simulink model "untitled"  (R2025a)
settings: Solver=VariableStepAuto  StartTime=0.0  StopTime=0.2  RelTol=1e-3
settings Model: Creator=vm66c  LastModifiedBy=vm66c

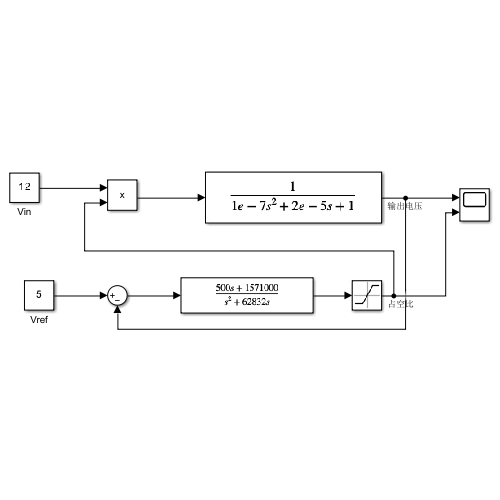
[thumbnail: Simulink's stored preview of the top-level diagram]
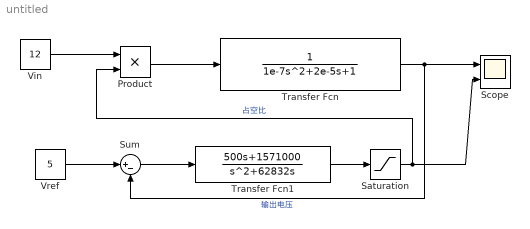
== system untitled ==
  Product : Product
  Saturation : Saturate  UpperLimit=0.9  LowerLimit=0.1
  Scope : Scope  NumInputPorts=2
      settings: ActiveDisplayYMinimum=-70.471139080263853  ActiveDisplayYMaximum=80.3935171752665
  Sum : Sum  Inputs=|+-
  Transfer Fcn : TransferFcn  Denominator=[1e-7, 2e-5, 1]
  Transfer Fcn1 : TransferFcn  Numerator=[500, 1571000]  Denominator=[1, 62832, 0]
  Vin : Constant  Value=12
  Vref : Constant  Value=5
  wires:
  Vin/1 -> Product/1
  Product/1 -> Transfer Fcn/1
  Vref/1 -> Sum/1
  Transfer Fcn/1 -> Scope/1, Sum/2  "输出电压"
  Sum/1 -> Transfer Fcn1/1
  Transfer Fcn1/1 -> Saturation/1
  Saturation/1 -> Product/2, Scope/2  "占空比"
